simulink model "SecRwRtStArmScrnTrgtPosSelc"  (R2018b)
settings: Solver=FixedStepDiscrete  StartTime=0.0  StopTime=10.0  FixedStep=0.01  RelTol=1e-3
undefined symbols (not defined in the file or in its folder): KeSMSw6sAcsEntrySecRwRtStArmScrnPos_Val, KeSMSw6sAcsEntrySecRwRtStArmScrnPosMax_Val, KeSMSw6sAcsEntrySecRwRtStArmScrnPosMin_Val, KeSMSw6sAcsExtSecRwRtStArmScrnPos_Val, KeSMSw6sAcsExtSecRwRtStArmScrnPosMax_Val, KeSMSw6sAcsExtSecRwRtStArmScrnPosMin_Val, KeSMSwAcsEntrySecRwRtStArmScrnPos_Val, KeSMSwAcsEntrySecRwRtStArmScrnPosMax_Val, KeSMSwAcsEntrySecRwRtStArmScrnPosMin_Val, KeSMSwAcsExtSecRwRtStArmScrnPos_Val, KeSMSwAcsExtSecRwRtStArmScrnPosMax_Val, KeSMSwAcsExtSecRwRtStArmScrnPosMin_Val
libraries: TrgtPosSelcLib x3
settings Model: Creator=sn2xws  LastModifiedBy=sn2xws
settings DataIOCC: SaveFormat=StructureWithTime
settings OptimizationCC: DefaultParameterBehavior=Inlined  EnhancedBackFolding=on  PassReuseOutputArgsAs=Individual arguments  ZeroExternalMemoryAtStartup=off  ZeroInternalMemoryAtStartup=off  OptimizeBlockOrder=speed  DifferentSizesBufferReuse=on  OptimizationCustomize=off
settings DebuggingCC: ParameterTunabilityLossMsg=error
settings ModelReferenceCC: ModelReferenceNumInstancesAllowed=Single
settings SFSimCC: MATLABDynamicMemAlloc=off
settings RTWCC: SystemTargetFile=autosar.tlc  GenCodeOnly=on  TemplateMakefile=ert_default_tmf  Description=AUTOSAR  GenerateReport=on  IncludeHyperlinkInReport=on  LaunchReport=on  GenerateTraceInfo=on  GenerateTraceReport=on  GenerateTraceReportSl=on  GenerateTraceReportSf=on  GenerateTraceReportEml=on
settings CodeAppCC: ForceParamTrailComments=on  IgnoreCustomStorageClasses=off  OperatorAnnotations=on  SimulinkDataObjDesc=on  SFDataObjDesc=on  InsertBlockDesc=on
settings STFCustomTargetCC: TargetLangStandard=C99 (ISO)  MultiwordLength=256  ParMdlRefBuildCompliant=on  CompOptLevelCompliant=on  IncludeMdlTerminateFcn=off  CombineOutputUpdateFcns=on  SuppressErrorStatus=on  ERTCustomFileBanners=on  SupportNonFinite=off  SupportComplex=off  SupportContinuousTime=off  SupportNonInlinedSFcns=off  RemoveResetFunc=on  MATLABClassNameForMDSCustomization=Simulink.SoftwareTarget.ERTCustomization  AutosarCompliant=on  UseToolchainInfoCompliant=on  LookupTableObjectStructAxisOrder=2,1,3,4,...  LUTObjectStructOrderEvenSpacing=Size,Table,Breakpoints  SystemTargetFile=autosar.tlc
settings ERTTargetCC: TargetLangStandard=C99 (ISO)  ConcurrentExecutionCompliant=off  IncludeMdlTerminateFcn=off  SuppressErrorStatus=on  SupportNonFinite=off  SupportComplex=off  ModelStepFunctionPrototypeControlCompliant=off  CPPClassGenCompliant=off  AutosarCompliant=on  LookupTableObjectStructAxisOrder=2,1,3,4,...  LUTObjectStructOrderEvenSpacing=Size,Table,Breakpoints  InlinedParameterPlacement=NonHierarchical  ERTCustomFileTemplate=example_file_process.tlc  ERTFilePackagingFormat=Compact

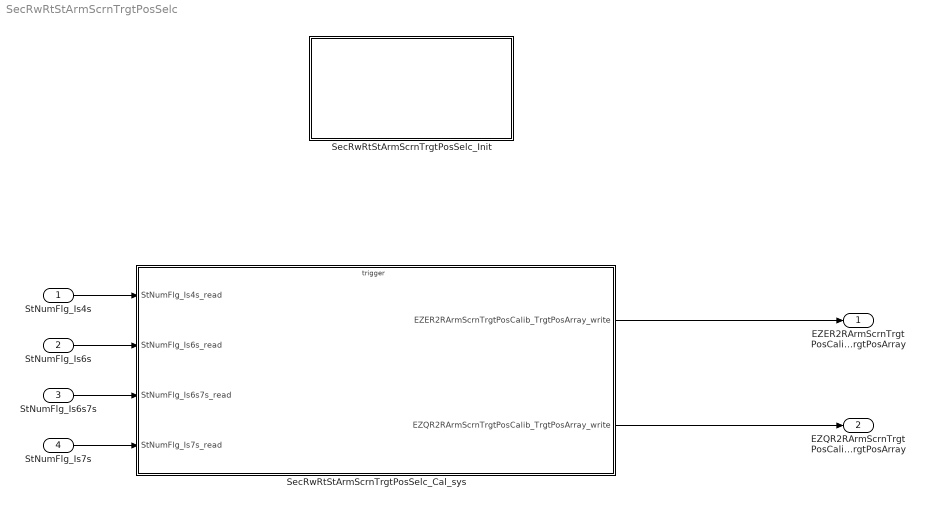
== system SecRwRtStArmScrnTrgtPosSelc ==
  StNumFlg_Is4s : Inport  OutDataTypeStr=boolean  PortDimensions=1
  StNumFlg_Is6s : Inport  Port=2  OutDataTypeStr=boolean  PortDimensions=1
  StNumFlg_Is6s7s : Inport  Port=3  OutDataTypeStr=boolean  PortDimensions=1
  StNumFlg_Is7s : Inport  Port=4  OutDataTypeStr=boolean  PortDimensions=1
  SecRwRtStArmScrnTrgtPosSelc_Cal_sys : Subsystem
  SecRwRtStArmScrnTrgtPosSelc_Init : Subsystem
  EZER2RArmScrnTrgtPosCalib_TrgtPosArray : Outport  Description=|  OutDataTypeStr=uint16  PortDimensions=3
      | 0:Pos
      | 1:Max
      | 2:Min
  EZQR2RArmScrnTrgtPosCalib_TrgtPosArray : Outport  Description=|  Port=2  OutDataTypeStr=uint16  PortDimensions=3
      | 0:Pos
      | 1:Max
      | 2:Min
  wires:
  StNumFlg_Is4s/1 -> SecRwRtStArmScrnTrgtPosSelc_Cal_sys/1(StNumFlg_Is4s_read)
  StNumFlg_Is6s/1 -> SecRwRtStArmScrnTrgtPosSelc_Cal_sys/2(StNumFlg_Is6s_read)
  StNumFlg_Is6s7s/1 -> SecRwRtStArmScrnTrgtPosSelc_Cal_sys/3(StNumFlg_Is6s7s_read)
  StNumFlg_Is7s/1 -> SecRwRtStArmScrnTrgtPosSelc_Cal_sys/4(StNumFlg_Is7s_read)
  SecRwRtStArmScrnTrgtPosSelc_Cal_sys/1(EZER2RArmScrnTrgtPosCalib_TrgtPosArray_write) -> EZER2RArmScrnTrgtPosCalib_TrgtPosArray/1
  SecRwRtStArmScrnTrgtPosSelc_Cal_sys/2(EZQR2RArmScrnTrgtPosCalib_TrgtPosArray_write) -> EZQR2RArmScrnTrgtPosCalib_TrgtPosArray/1

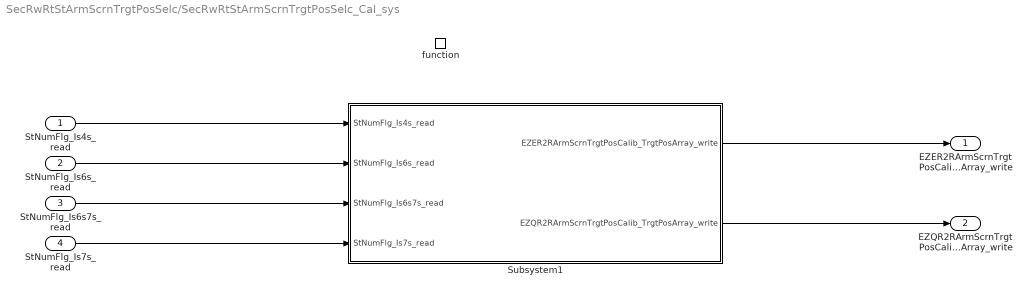
== system SecRwRtStArmScrnTrgtPosSelc/SecRwRtStArmScrnTrgtPosSelc_Cal_sys ==
  StNumFlg_Is4s_read : Inport
  StNumFlg_Is6s_read : Inport  Port=2
  StNumFlg_Is6s7s_read : Inport  Port=3
  StNumFlg_Is7s_read : Inport  Port=4
  function : TriggerPort  TriggerType=function-call  IsSimulinkFunction=on  FunctionName=SecRwRtStArmScrnTrgtPosSelc_Cal  VariantControl=(inherit)
  Subsystem1 : Subsystem
  EZER2RArmScrnTrgtPosCalib_TrgtPosArray_write : Outport
      settings: EnsureOutportIsVirtual=on
  EZQR2RArmScrnTrgtPosCalib_TrgtPosArray_write : Outport  Port=2
      settings: EnsureOutportIsVirtual=on
  wires:
  StNumFlg_Is4s_read/1 -> Subsystem1/1(StNumFlg_Is4s_read)
  StNumFlg_Is6s_read/1 -> Subsystem1/2(StNumFlg_Is6s_read)
  StNumFlg_Is6s7s_read/1 -> Subsystem1/3(StNumFlg_Is6s7s_read)
  StNumFlg_Is7s_read/1 -> Subsystem1/4(StNumFlg_Is7s_read)
  Subsystem1/1(EZER2RArmScrnTrgtPosCalib_TrgtPosArray_write) -> EZER2RArmScrnTrgtPosCalib_TrgtPosArray_write/1
  Subsystem1/2(EZQR2RArmScrnTrgtPosCalib_TrgtPosArray_write) -> EZQR2RArmScrnTrgtPosCalib_TrgtPosArray_write/1

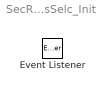
== system SecRwRtStArmScrnTrgtPosSelc/SecRwRtStArmScrnTrgtPosSelc_Init ==
  Event Listener : EventListener  EventName=reset

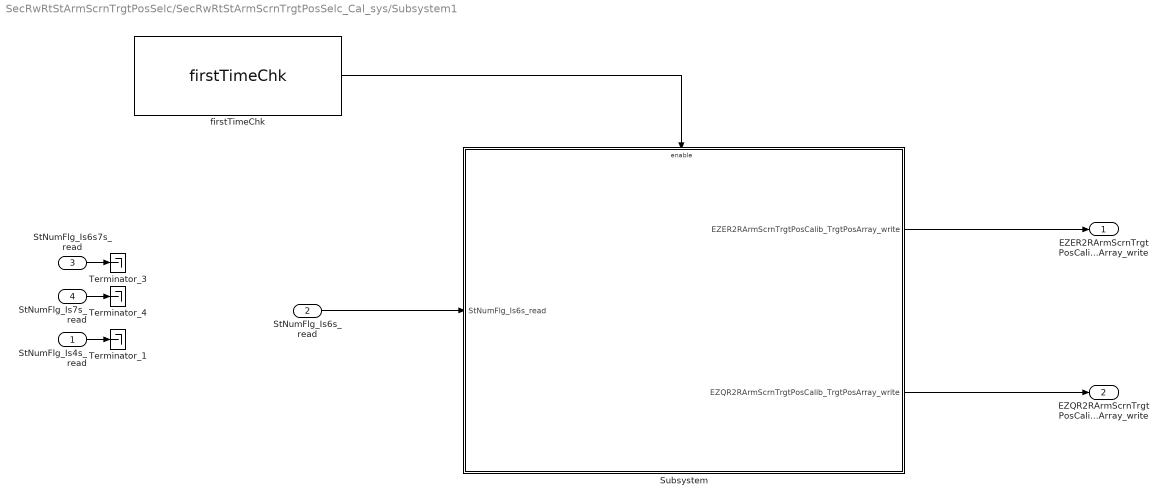
== system SecRwRtStArmScrnTrgtPosSelc/SecRwRtStArmScrnTrgtPosSelc_Cal_sys/Subsystem1 ==
  StNumFlg_Is4s_read : Inport
  StNumFlg_Is6s_read : Inport  Port=2
  StNumFlg_Is6s7s_read : Inport  Port=3
  StNumFlg_Is7s_read : Inport  Port=4
  Subsystem : Subsystem
  Terminator_1 : Terminator
  Terminator_3 : Terminator
  Terminator_4 : Terminator
  firstTimeChk : TrgtPosSelcLib/firstTimeChk  SystemSampleTime=-1
  EZER2RArmScrnTrgtPosCalib_TrgtPosArray_write : Outport
      settings: EnsureOutportIsVirtual=on
  EZQR2RArmScrnTrgtPosCalib_TrgtPosArray_write : Outport  Port=2
      settings: EnsureOutportIsVirtual=on
  wires:
  StNumFlg_Is6s7s_read/1 -> Terminator_3/1
  StNumFlg_Is4s_read/1 -> Terminator_1/1
  StNumFlg_Is7s_read/1 -> Terminator_4/1
  Subsystem/2(EZQR2RArmScrnTrgtPosCalib_TrgtPosArray_write) -> EZQR2RArmScrnTrgtPosCalib_TrgtPosArray_write/1
  Subsystem/1(EZER2RArmScrnTrgtPosCalib_TrgtPosArray_write) -> EZER2RArmScrnTrgtPosCalib_TrgtPosArray_write/1
  firstTimeChk/1 -> Subsystem/Enable
  StNumFlg_Is6s_read/1 -> Subsystem/1(StNumFlg_Is6s_read)

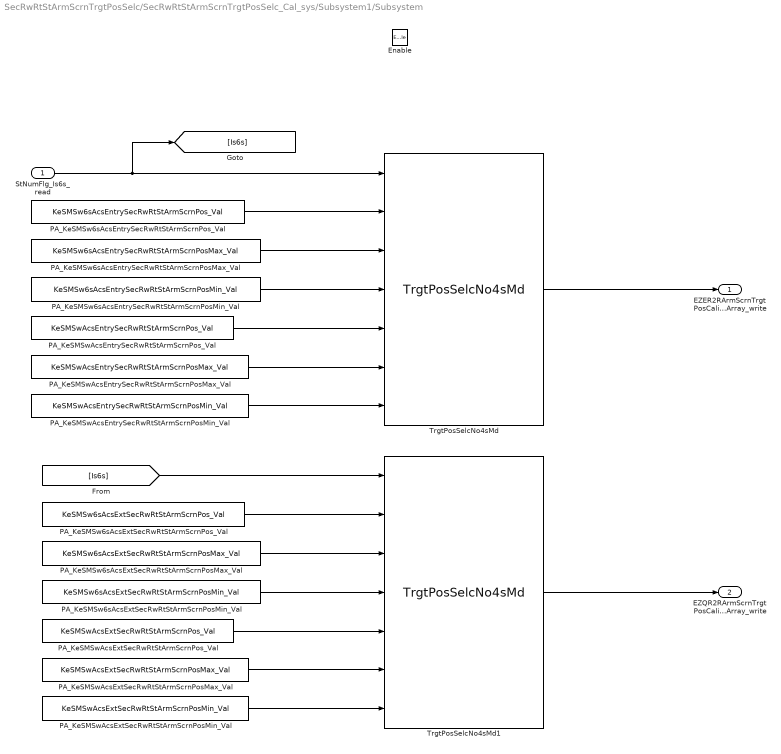
== system SecRwRtStArmScrnTrgtPosSelc/SecRwRtStArmScrnTrgtPosSelc_Cal_sys/Subsystem1/Subsystem ==
  StNumFlg_Is6s_read : Inport
  Enable : EnablePort
  PA_KeSMSw6sAcsEntrySecRwRtStArmScrnPosMax_Val : Constant  Value=KeSMSw6sAcsEntrySecRwRtStArmScrnPosMax_Val
  PA_KeSMSw6sAcsEntrySecRwRtStArmScrnPosMin_Val : Constant  Value=KeSMSw6sAcsEntrySecRwRtStArmScrnPosMin_Val
  PA_KeSMSw6sAcsEntrySecRwRtStArmScrnPos_Val : Constant  Value=KeSMSw6sAcsEntrySecRwRtStArmScrnPos_Val
  PA_KeSMSw6sAcsExtSecRwRtStArmScrnPosMax_Val : Constant  Value=KeSMSw6sAcsExtSecRwRtStArmScrnPosMax_Val
  PA_KeSMSw6sAcsExtSecRwRtStArmScrnPosMin_Val : Constant  Value=KeSMSw6sAcsExtSecRwRtStArmScrnPosMin_Val
  PA_KeSMSw6sAcsExtSecRwRtStArmScrnPos_Val : Constant  Value=KeSMSw6sAcsExtSecRwRtStArmScrnPos_Val
  PA_KeSMSwAcsEntrySecRwRtStArmScrnPosMax_Val : Constant  Value=KeSMSwAcsEntrySecRwRtStArmScrnPosMax_Val
  PA_KeSMSwAcsEntrySecRwRtStArmScrnPosMin_Val : Constant  Value=KeSMSwAcsEntrySecRwRtStArmScrnPosMin_Val
  PA_KeSMSwAcsEntrySecRwRtStArmScrnPos_Val : Constant  Value=KeSMSwAcsEntrySecRwRtStArmScrnPos_Val
  PA_KeSMSwAcsExtSecRwRtStArmScrnPosMax_Val : Constant  Value=KeSMSwAcsExtSecRwRtStArmScrnPosMax_Val
  PA_KeSMSwAcsExtSecRwRtStArmScrnPosMin_Val : Constant  Value=KeSMSwAcsExtSecRwRtStArmScrnPosMin_Val
  PA_KeSMSwAcsExtSecRwRtStArmScrnPos_Val : Constant  Value=KeSMSwAcsExtSecRwRtStArmScrnPos_Val
  TrgtPosSelcNo4sMd : TrgtPosSelcLib/TrgtPosSelcNo4sMd  SystemSampleTime=-1
  TrgtPosSelcNo4sMd1 : TrgtPosSelcLib/TrgtPosSelcNo4sMd  SystemSampleTime=-1
  EZER2RArmScrnTrgtPosCalib_TrgtPosArray_write : Outport
      settings: EnsureOutportIsVirtual=on
  EZQR2RArmScrnTrgtPosCalib_TrgtPosArray_write : Outport  Port=2
      settings: EnsureOutportIsVirtual=on
  wires:
  PA_KeSMSw6sAcsExtSecRwRtStArmScrnPos_Val/1 -> TrgtPosSelcNo4sMd1/2
  StNumFlg_Is6s_read/1 -> [Is6s], TrgtPosSelcNo4sMd/1
  TrgtPosSelcNo4sMd/1 -> EZER2RArmScrnTrgtPosCalib_TrgtPosArray_write/1
  PA_KeSMSw6sAcsEntrySecRwRtStArmScrnPos_Val/1 -> TrgtPosSelcNo4sMd/2
  PA_KeSMSw6sAcsEntrySecRwRtStArmScrnPosMax_Val/1 -> TrgtPosSelcNo4sMd/3
  PA_KeSMSw6sAcsEntrySecRwRtStArmScrnPosMin_Val/1 -> TrgtPosSelcNo4sMd/4
  TrgtPosSelcNo4sMd1/1 -> EZQR2RArmScrnTrgtPosCalib_TrgtPosArray_write/1
  PA_KeSMSwAcsExtSecRwRtStArmScrnPos_Val/1 -> TrgtPosSelcNo4sMd1/5
  PA_KeSMSwAcsExtSecRwRtStArmScrnPosMax_Val/1 -> TrgtPosSelcNo4sMd1/6
  PA_KeSMSwAcsExtSecRwRtStArmScrnPosMin_Val/1 -> TrgtPosSelcNo4sMd1/7
  PA_KeSMSw6sAcsExtSecRwRtStArmScrnPosMax_Val/1 -> TrgtPosSelcNo4sMd1/3
  PA_KeSMSw6sAcsExtSecRwRtStArmScrnPosMin_Val/1 -> TrgtPosSelcNo4sMd1/4
  PA_KeSMSwAcsEntrySecRwRtStArmScrnPos_Val/1 -> TrgtPosSelcNo4sMd/5
  PA_KeSMSwAcsEntrySecRwRtStArmScrnPosMax_Val/1 -> TrgtPosSelcNo4sMd/6
  PA_KeSMSwAcsEntrySecRwRtStArmScrnPosMin_Val/1 -> TrgtPosSelcNo4sMd/7
  [Is6s] -> TrgtPosSelcNo4sMd1/1
